simulink model "MOBATSim"  (R2021a)
settings: Solver=FixedStepAuto  StartTime=0.0  StopTime=Sim_t  FixedStep=0.01  MinStep=0.01  RelTol=1e-2
undefined symbols (not defined in the file): meters, Sim_Ts, Vehicle_id, Vehicles
libraries: simulink x31, robotalgslib x11, drivingvehiclecontroller x11, mpcadaslib x1, pid_lib x1
(part 1 of 5)
Description:
  | MOBATSim (Model-based Autonomous Traffic Simulation Framework) is a simulation framework based on MATLAB and Simulink that allows users to develop automated driving algorithms to assess their safety and performance. By running a traffic simulation, the safety of the implemented component or algorithm is measured on both the vehicle level and the traffic level, supported by 2D and 3D visualization options.
settings Model: VariantFading=off  Creator=Mustafa  LastModifiedBy=RanGreidi
settings SolverCC: AlgebraicLoopSolver=TrustRegion  AutoInsertRateTranBlk=on  InsertRTBMode=Always  MinimalZcImpactIntegration=on
settings DataIOCC: ReturnWorkspaceOutputs=off
settings DebuggingCC: AlgebraicLoopMsg=error  UniqueDataStoreMsg=error  SFMachineParentedDataDiag=warning  ArithmeticOperatorsInVariantConditions=warning
settings SFSimCC: SimUseLocalCustomCode=off  CustomCodeUndefinedFunction=UseInterfaceOnly
settings RTWCC: RTWUseLocalCustomCode=off
settings CodeAppCC: StateflowObjectComments=on

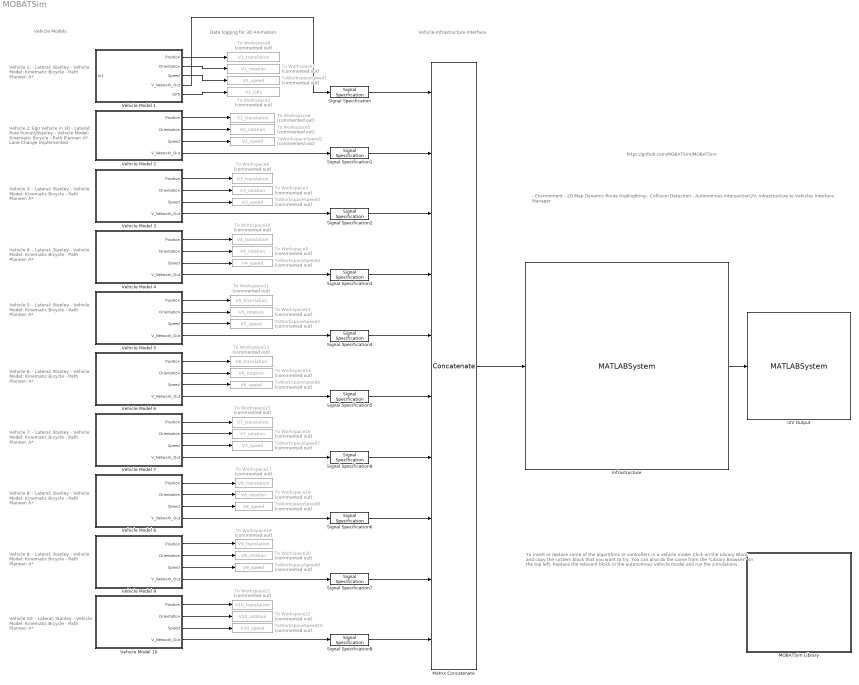
== system MOBATSim ==
  note: Vehicle 1:
      | - Lateral: Stanley
      | - Vehicle Model: Kinematic Bicycle
      | - Path Planner: A*
  note: https://github.com/MOBATSim/MOBATSim
  note: To insert or replace some of the algorithms
      | or controllers in a vehicle mode:
      | Click on the Library Block and copy the system block that you want to try. You can also do the same from the "Library Browser" on the top left.
      | Replace the relevant block in the autonomous vehicle model and run the simulations.
  note: Data logging for 3D Animation
  note: Vehicle-Infrastructure Interface
  note: Vehicle 2: Ego Vehicle in 3D
      | - Lateral: Pure Pursuit/Stanley
      | - Vehicle Model: Kinematic Bicycle
      | - Path Planner: A*
      | - Lane Change Implemented
  note: Vehicle 3:
      | - Lateral: Stanley
      | - Vehicle Model: Kinematic Bicycle
      | - Path Planner: A*
  note: Vehicle 4:
      | - Lateral: Stanley
      | - Vehicle Model: Kinematic Bicycle
      | - Path Planner: A*
  note: Vehicle 6:
      | - Lateral: Stanley
      | - Vehicle Model: Kinematic Bicycle
      | - Path Planner: A*
  note: Vehicle 7:
      | - Lateral: Stanley
      | - Vehicle Model: Kinematic Bicycle
      | - Path Planner: A*
  note: Vehicle 8:
      | - Lateral: Stanley
      | - Vehicle Model: Kinematic Bicycle
      | - Path Planner: A*
  note: Vehicle 9:
      | - Lateral: Stanley
      | - Vehicle Model: Kinematic Bicycle
      | - Path Planner: A*
  note: Vehicle 10:
      | - Lateral: Stanley
      | - Vehicle Model: Kinematic Bicycle
      | - Path Planner: A*
  note: Vehicle 5:
      | - Lateral: Stanley
      | - Vehicle Model: Kinematic Bicycle
      | - Path Planner: A*
  note: Vehicle Models
  note: I2V: Infrastructure to Vehicles Interface
  note: - Environment
      | - 2D Map Dynamic Route Highlighting
      | - Collision Detection
      | - Autonomous Intersection Manager
  I2V Output : MATLABSystem  System=I2V  SimulateUsing=Interpreted execution
      mask Type: I2V
      mask Display:
      | image('MOBATSIM-Icon-Set_3- Flags.png');
      | port_label('input',1,'Flags');
  Infrastructure : MATLABSystem  Description=An instance of the Map.m Class is created.  System=Infrastructure  nrVehicles=length(Vehicles)  SimulateUsing=Interpreted execution
      mask Type: Infrastructure
      mask Display:
      | image('MOBATSIM-Icon-Set_5- Intersection.png');
      | port_label('input',1,'V2Idata');
      | port_label('output',1,'StopCommands');
  MOBATSim Library : Subsystem
      mask Display: image('$imagefile'); % Use "Edit Image" on toolstrip to change.
  Matrix Concatenate : Concatenate  NumInputs=10  Mode=Multidimensional array
  Signal Specification{,1..9} (10 alike) : SignalSpecification  Dimensions=[1 2]
  To Workspace1 : ToWorkspace  Commented=on  VariableName=V1_GPS  SaveFormat=Timeseries  SampleTime=-1
  To Workspace10 : ToWorkspace  Commented=on  VariableName=V4_translation  SaveFormat=Timeseries  SampleTime=-1
  To Workspace11 : ToWorkspace  Commented=on  VariableName=V5_translation  SaveFormat=Timeseries  SampleTime=-1
  To Workspace12 : ToWorkspace  Commented=on  VariableName=V5_rotation  SaveFormat=Timeseries  SampleTime=-1
  To Workspace13 : ToWorkspace  Commented=on  VariableName=V6_translation  SaveFormat=Timeseries  SampleTime=-1
  To Workspace14 : ToWorkspace  Commented=on  VariableName=V6_rotation  SaveFormat=Timeseries  SampleTime=-1
  To Workspace15 : ToWorkspace  Commented=on  VariableName=V7_translation  SaveFormat=Timeseries  SampleTime=-1
  To Workspace16 : ToWorkspace  Commented=on  VariableName=V7_rotation  SaveFormat=Timeseries  SampleTime=-1
  To Workspace17 : ToWorkspace  Commented=on  VariableName=V8_translation  SaveFormat=Timeseries  SampleTime=-1
  To Workspace18 : ToWorkspace  Commented=on  VariableName=V8_rotation  SaveFormat=Timeseries  SampleTime=-1
  To Workspace19 : ToWorkspace  Commented=on  VariableName=V9_translation  SaveFormat=Timeseries  SampleTime=-1
  To Workspace20 : ToWorkspace  Commented=on  VariableName=V9_rotation  SaveFormat=Timeseries  SampleTime=-1
  To Workspace21 : ToWorkspace  Commented=on  VariableName=V10_translation  SaveFormat=Timeseries  SampleTime=-1
  To Workspace22 : ToWorkspace  Commented=on  VariableName=V10_rotation  SaveFormat=Timeseries  SampleTime=-1
  To Workspace3 : ToWorkspace  Commented=on  VariableName=V3_rotation  SaveFormat=Timeseries  SampleTime=-1
  To Workspace4 : ToWorkspace  Commented=on  VariableName=V3_translation  SaveFormat=Timeseries  SampleTime=-1
  To Workspace5 : ToWorkspace  Commented=on  VariableName=V2_rotation  SaveFormat=Timeseries  SampleTime=-1
  To Workspace6 : ToWorkspace  Commented=on  VariableName=V2_translation  SaveFormat=Timeseries  SampleTime=-1
  To Workspace7 : ToWorkspace  Commented=on  VariableName=V1_rotation  SaveFormat=Timeseries  SampleTime=-1
  To Workspace8 : ToWorkspace  Commented=on  VariableName=V1_translation  SaveFormat=Timeseries  SampleTime=-1
  To Workspace9 : ToWorkspace  Commented=on  VariableName=V4_rotation  SaveFormat=Timeseries  SampleTime=-1
  ToWorkspaceSpeed1 : ToWorkspace  Commented=on  VariableName=V1_speed  SaveFormat=Timeseries  SampleTime=-1
  ToWorkspaceSpeed10 : ToWorkspace  Commented=on  VariableName=V10_speed  SaveFormat=Timeseries  SampleTime=-1
  ToWorkspaceSpeed2 : ToWorkspace  Commented=on  VariableName=V2_speed  SaveFormat=Timeseries  SampleTime=-1
  "ToWorkspaceSpeed3 " : ToWorkspace  Commented=on  VariableName=V3_speed  SaveFormat=Timeseries  SampleTime=-1
  ToWorkspaceSpeed4 : ToWorkspace  Commented=on  VariableName=V4_speed  SaveFormat=Timeseries  SampleTime=-1
  ToWorkspaceSpeed5 : ToWorkspace  Commented=on  VariableName=V5_speed  SaveFormat=Timeseries  SampleTime=-1
  ToWorkspaceSpeed6 : ToWorkspace  Commented=on  VariableName=V6_speed  SaveFormat=Timeseries  SampleTime=-1
  ToWorkspaceSpeed7 : ToWorkspace  Commented=on  VariableName=V7_speed  SaveFormat=Timeseries  SampleTime=-1
  ToWorkspaceSpeed8 : ToWorkspace  Commented=on  VariableName=V8_speed  SaveFormat=Timeseries  SampleTime=-1
  ToWorkspaceSpeed9 : ToWorkspace  Commented=on  VariableName=V9_speed  SaveFormat=Timeseries  SampleTime=-1
  Vehicle Model 1 : Subsystem  Description=Tag: Autonomous Vehicle Model  SystemSampleTime=0.01  mask{Vehicle_id=1}
      mask TypeOptions Vehicle_id: MATLAB System2/Vehicle_id
      mask DialogControl DescTextVar Prompt: Autonomous Vehicle Model defined as a system, press the arrow on the lower left corner to see the subsystems. The initial parameters below should be taken from the base workspace but you can edit them anyway you like.
      mask Display: image('$imagefile'); % Use "Edit Image" on toolstrip to change.
  Vehicle Model 10 : Subsystem  Description=Tag: Autonomous Vehicle Model  SystemSampleTime=0.01  mask{Vehicle_id=10}
      mask TypeOptions Vehicle_id: MATLAB System2/Vehicle_id
      mask DialogControl DescTextVar Prompt: Autonomous Vehicle Model defined as a system, press the arrow on the lower left corner to see the subsystems. The initial parameters below should be taken from the base workspace but you can edit them anyway you like.
      mask Display: image('$imagefile'); % Use "Edit Image" on toolstrip to change.
  Vehicle Model 2 : Subsystem  Description=Tag: Autonomous Vehicle Model  SystemSampleTime=0.01  mask{Vehicle_id=2}
      mask TypeOptions Vehicle_id: MATLAB System2/Vehicle_id
      mask DialogControl DescTextVar Prompt: Autonomous Vehicle Model defined as a system, press the arrow on the lower left corner to see the subsystems. The initial parameters below should be taken from the base workspace but you can edit them anyway you like.
      mask Display: image('$imagefile'); % Use "Edit Image" on toolstrip to change.
  Vehicle Model 3 : Subsystem  Description=Tag: Autonomous Vehicle Model  SystemSampleTime=0.01  mask{Vehicle_id=3}
      mask TypeOptions Vehicle_id: MATLAB System2/Vehicle_id
      mask DialogControl DescTextVar Prompt: Autonomous Vehicle Model defined as a system, press the arrow on the lower left corner to see the subsystems. The initial parameters below should be taken from the base workspace but you can edit them anyway you like.
      mask Display: image('$imagefile'); % Use "Edit Image" on toolstrip to change.
  Vehicle Model 4 : Subsystem  Description=Tag: Autonomous Vehicle Model  SystemSampleTime=0.01  mask{Vehicle_id=4}
      mask TypeOptions Vehicle_id: MATLAB System2/Vehicle_id
      mask DialogControl DescTextVar Prompt: Autonomous Vehicle Model defined as a system, press the arrow on the lower left corner to see the subsystems. The initial parameters below should be taken from the base workspace but you can edit them anyway you like.
      mask Display: image('$imagefile'); % Use "Edit Image" on toolstrip to change.
  Vehicle Model 5 : Subsystem  Description=Tag: Autonomous Vehicle Model  SystemSampleTime=0.01  mask{Vehicle_id=5}
      mask TypeOptions Vehicle_id: MATLAB System2/Vehicle_id
      mask DialogControl DescTextVar Prompt: Autonomous Vehicle Model defined as a system, press the arrow on the lower left corner to see the subsystems. The initial parameters below should be taken from the base workspace but you can edit them anyway you like.
      mask Display: image('$imagefile'); % Use "Edit Image" on toolstrip to change.
  Vehicle Model 6 : Subsystem  Description=Tag: Autonomous Vehicle Model  SystemSampleTime=0.01  mask{Vehicle_id=6}
      mask TypeOptions Vehicle_id: MATLAB System2/Vehicle_id
      mask DialogControl DescTextVar Prompt: Autonomous Vehicle Model defined as a system, press the arrow on the lower left corner to see the subsystems. The initial parameters below should be taken from the base workspace but you can edit them anyway you like.
      mask Display: image('$imagefile'); % Use "Edit Image" on toolstrip to change.
  Vehicle Model 7 : Subsystem  Description=Tag: Autonomous Vehicle Model  SystemSampleTime=0.01  mask{Vehicle_id=7}
      mask TypeOptions Vehicle_id: MATLAB System2/Vehicle_id
      mask DialogControl DescTextVar Prompt: Autonomous Vehicle Model defined as a system, press the arrow on the lower left corner to see the subsystems. The initial parameters below should be taken from the base workspace but you can edit them anyway you like.
      mask Display: image('$imagefile'); % Use "Edit Image" on toolstrip to change.
  Vehicle Model 8 : Subsystem  Description=Tag: Autonomous Vehicle Model  SystemSampleTime=0.01  mask{Vehicle_id=8}
      mask TypeOptions Vehicle_id: MATLAB System2/Vehicle_id
      mask DialogControl DescTextVar Prompt: Autonomous Vehicle Model defined as a system, press the arrow on the lower left corner to see the subsystems. The initial parameters below should be taken from the base workspace but you can edit them anyway you like.
      mask Display: image('$imagefile'); % Use "Edit Image" on toolstrip to change.
  Vehicle Model 9 : Subsystem  Description=Tag: Autonomous Vehicle Model  SystemSampleTime=0.01  mask{Vehicle_id=9}
      mask TypeOptions Vehicle_id: MATLAB System2/Vehicle_id
      mask DialogControl DescTextVar Prompt: Autonomous Vehicle Model defined as a system, press the arrow on the lower left corner to see the subsystems. The initial parameters below should be taken from the base workspace but you can edit them anyway you like.
      mask Display: image('$imagefile'); % Use "Edit Image" on toolstrip to change.
  wires:
  Vehicle Model 1/1(Position) -> To Workspace8/1
  Vehicle Model 1/2(Orientation) -> To Workspace7/1
  Vehicle Model 1/4(V_Network_Out) -> Signal Specification/1
  Signal Specification/1 -> Matrix Concatenate/1
  Signal Specification1/1 -> Matrix Concatenate/2
  Vehicle Model 2/2(Orientation) -> To Workspace5/1
  Vehicle Model 2/1(Position) -> To Workspace6/1
  Vehicle Model 3/2(Orientation) -> To Workspace3/1
  Vehicle Model 3/1(Position) -> To Workspace4/1
  Signal Specification2/1 -> Matrix Concatenate/3
  Infrastructure/1 -> I2V Output/1
  Vehicle Model 8/4(V_Network_Out) -> Signal Specification6/1
  Vehicle Model 9/4(V_Network_Out) -> Signal Specification7/1
  Vehicle Model 10/4(V_Network_Out) -> Signal Specification8/1
  Signal Specification3/1 -> Matrix Concatenate/4
  Signal Specification4/1 -> Matrix Concatenate/5
  Signal Specification5/1 -> Matrix Concatenate/6
  Signal Specification9/1 -> Matrix Concatenate/7
  Signal Specification6/1 -> Matrix Concatenate/8
  Signal Specification7/1 -> Matrix Concatenate/9
  Signal Specification8/1 -> Matrix Concatenate/10
  Vehicle Model 4/2(Orientation) -> To Workspace9/1
  Vehicle Model 4/1(Position) -> To Workspace10/1
  Vehicle Model 6/2(Orientation) -> To Workspace14/1
  Vehicle Model 6/1(Position) -> To Workspace13/1
  Vehicle Model 7/2(Orientation) -> To Workspace16/1
  Vehicle Model 7/1(Position) -> To Workspace15/1
  Vehicle Model 8/2(Orientation) -> To Workspace18/1
  Vehicle Model 8/1(Position) -> To Workspace17/1
  Vehicle Model 9/2(Orientation) -> To Workspace20/1
  Vehicle Model 9/1(Position) -> To Workspace19/1
  Vehicle Model 10/2(Orientation) -> To Workspace22/1
  Vehicle Model 10/1(Position) -> To Workspace21/1
  Matrix Concatenate/1 -> Infrastructure/1
  Vehicle Model 2/4(V_Network_Out) -> Signal Specification1/1
  Vehicle Model 3/4(V_Network_Out) -> Signal Specification2/1
  Vehicle Model 4/4(V_Network_Out) -> Signal Specification3/1
  Vehicle Model 6/4(V_Network_Out) -> Signal Specification5/1
  Vehicle Model 7/4(V_Network_Out) -> Signal Specification9/1
  Vehicle Model 5/1(Position) -> To Workspace11/1
  Vehicle Model 5/2(Orientation) -> To Workspace12/1
  Vehicle Model 5/4(V_Network_Out) -> Signal Specification4/1
  Vehicle Model 1/3(Speed) -> ToWorkspaceSpeed1/1
  Vehicle Model 2/3(Speed) -> ToWorkspaceSpeed2/1
  Vehicle Model 3/3(Speed) -> "ToWorkspaceSpeed3 "/1
  Vehicle Model 4/3(Speed) -> ToWorkspaceSpeed4/1
  Vehicle Model 5/3(Speed) -> ToWorkspaceSpeed5/1
  Vehicle Model 6/3(Speed) -> ToWorkspaceSpeed6/1
  Vehicle Model 7/3(Speed) -> ToWorkspaceSpeed7/1
  Vehicle Model 8/3(Speed) -> ToWorkspaceSpeed8/1
  Vehicle Model 9/3(Speed) -> ToWorkspaceSpeed9/1
  Vehicle Model 10/3(Speed) -> ToWorkspaceSpeed10/1
  Vehicle Model 1/5(GPS) -> To Workspace1/1

== system MOBATSim/MOBATSim Library ==
  note: Different pathplanner algorithms with the same input/outputs. Some details and computational performances may differ.
  note: The ACC Classical Block from the MathWorks Example:
      | https://www.mathworks.com/help/driving/examples/adaptive-cruise-control-with-sensor-fusion.html
  note: Path Planners - MATLAB System Blocks
  note: Platoon Controllers - Subsystem Blocks
  note: Platoon controller-PID with a safe distance controller for safely following the
      | leading vehicle. Most vehicles have this block because it is simple and fast
      | in terms of execution time. Can be tuned.
  note: Standard MPC - Adaptive Cruise Control Block. Safest option but computationally
      | expensive. Tradeoff between safety and computational performance depends on
      | the prediction horizon variable.
  note: Lateral Controllers with MATLAB System Blocks
  ACC Classical : Subsystem  Commented=on  TreatAsAtomicUnit=on  VariantControl=controller_type == 1
      settings: RTWFileNameOpts=Use function name
  Adaptive Cruise Control System : mpcadaslib/Adaptive Cruise Control System  Commented=on  EgoModel=tf(1,[1,0])  InitialEgoVelocity=0  DefaultSpacing=Vehicles(Vehicle_id).sensors.safeDistance  MaxVelocity=Vehicles(Vehicle_id).dynamics.maxSpeed  MinAcceleration=-3  amin_ext=off  MaxAcceleration=2  amax_ext=off  Ts=0.1  PredictionHorizon=100  ControllerBehavior=0.620  suboptimal=off  maxiter=10  datatypeopt=double  optmode=off  trackmode=off
  Path Planner - AStar : MATLABSystem  Commented=on  System=VehiclePathPlanner_Astar  Vehicle_id=Vehicle_id  SimulateUsing=Interpreted execution
      mask Type: VehiclePathPlanner_Astar
      mask Display:
      | image('MOBATSIM-Icon-Set_8- Navigation.png');
      | port_label('input',1,'CommunicationIDs');
      | port_label('output',1,'waypointReached');
  Path Planner - Shortest : MATLABSystem  Commented=on  System=VehiclePathPlanner_shortestPathFinder  Vehicle_id=Vehicle_id  SimulateUsing=Interpreted execution
      mask Type: VehiclePathPlanner_shortestPathFinder
      mask Display:
      | image('MOBATSIM-Icon-Set_8- Navigation.png');
      | port_label('input',1,'CommunicationIDs');
      | port_label('output',1,'waypointReached');
  Platoon Controller - PID : Subsystem  Commented=on
  Pure Pursuit with Lane Changing : Subsystem  Commented=on
  Stanley Lateral Control : Subsystem  Commented=on

== system MOBATSim/Vehicle Model 1 ==
  note: Perception
  note: Decision-Making
  note: Control
  In1 : Inport
  Behavioural Planner : MATLABSystem  System=VehicleDrivingMode  Vehicle_id=Vehicle_id  SimulateUsing=Interpreted execution
      mask Type: VehicleDrivingMode
      mask Display:
      | image('MOBATSIM-Icon-Set_7- Behavioural Planner.png');
      | port_label('input',1,'vehicleDetected');
      | port_label('output',1,'SpeedReference');
      | port_label('output',2,'DistanceReference');
      | port_label('output',3,'LeadSpeed');
      | port_label('output',4,'DrivingMode');
      | port_label('output',5,'Dist2Stop');
      | port_label('output',6,'laneChange');
  From Workspace : FromWorkspace  VariableName=Vehicles(1,1).dynamics.GPS  SampleTime=0.02
  Longitudinal and Lateral Controllers : Subsystem
  Safety Filter : Subsystem
  Transform to MOBATSim Coordinates : Subsystem
  Vehicle Model - Kinematic 3DOF Single Track : Subsystem  mask{Vehicle_id=Vehicle_id}
      mask prompts: Vehicle_id "Vehicle ID"
      mask Display: image('MOBATSIM-Icon-Set_13- VehicleModel.png'); % Use "Edit Image" on toolstrip to change.
  Vehicle Path Planner : MATLABSystem  System=VehiclePathPlanner_Astar  Vehicle_id=Vehicle_id  SimulateUsing=Interpreted execution
      mask Type: VehiclePathPlanner_Astar
      mask Display:
      | image('MOBATSIM-Icon-Set_8- Navigation.png');
      | port_label('input',1,'CommunicationIDs');
      | port_label('output',1,'waypointReached');
  Vehicle Sensors : MATLABSystem  System=VehicleSensors  Vehicle_id=Vehicle_id  Tsample=Sim_Ts  OffsetTime=0  SimulateUsing=Interpreted execution
      mask Type: VehicleSensors
      mask Display:
      | image('MOBATSIM-Icon-Set_4- Sensor.png');
      | port_label('output',1,'V2VcommIDs');
      | port_label('output',2,'vehicleDetected');
  Vehicle V2I Output : MATLABSystem  System=VehicleV2I_Out  Vehicle_id=Vehicle_id  SimulateUsing=Interpreted execution
      mask Type: VehicleV2I_Out
      mask Display:
      | image('MOBATSIM-Icon-Set_6- V2l.png');
      | port_label('input',1,'waypointReached');
      | port_label('output',1,'V2Idata');
  Position : Outport  VectorParamsAs1DForOutWhenUnconnected=off
  Orientation : Outport  Port=2  VectorParamsAs1DForOutWhenUnconnected=off
  Speed : Outport  Port=3  VectorParamsAs1DForOutWhenUnconnected=off
  V_Network_Out : Outport  Port=4  VectorParamsAs1DForOutWhenUnconnected=off
  GPS : Outport  Port=5  VectorParamsAs1DForOutWhenUnconnected=off
  wires:
  Vehicle Path Planner/1 -> Vehicle V2I Output/1
  Vehicle Sensors/1 -> Vehicle Path Planner/1
  Vehicle V2I Output/1 -> V_Network_Out/1
  Vehicle Sensors/2 -> Behavioural Planner/1
  Behavioural Planner/1 -> Longitudinal and Lateral Controllers/1(Speed Reference)
  Behavioural Planner/2 -> Longitudinal and Lateral Controllers/2(Inter Vehicular Distance)
  Behavioural Planner/3 -> Longitudinal and Lateral Controllers/3(Lead Speed)
  Behavioural Planner/4 -> Longitudinal and Lateral Controllers/4(drivingMode)
  Behavioural Planner/5 -> Longitudinal and Lateral Controllers/5(Dist2Stop)
  Transform to MOBATSim Coordinates/1(Position) -> Position/1
  Transform to MOBATSim Coordinates/2(Orientation) -> Orientation/1
  Vehicle Model - Kinematic 3DOF Single Track/2(xdot) -> Longitudinal and Lateral Controllers/7(Actual Speed), Speed/1
  Vehicle Model - Kinematic 3DOF Single Track/1(Pose) -> Longitudinal and Lateral Controllers/8(Actual Pose), Transform to MOBATSim Coordinates/1(Pose)
  Longitudinal and Lateral Controllers/1(ref Acc) -> Safety Filter/1(Reference Acceleration)
  Longitudinal and Lateral Controllers/2(ref Steering) -> Safety Filter/2(Reference Steering Angle)
  Safety Filter/1(Steering Angle Cmd) -> Vehicle Model - Kinematic 3DOF Single Track/1(WhlAngF)
  Safety Filter/2(Speed_input) -> Vehicle Model - Kinematic 3DOF Single Track/2(xdotin)
  Behavioural Planner/6 -> Longitudinal and Lateral Controllers/6(laneChange)
  From Workspace/1 -> ?

== system MOBATSim/Vehicle Model 10 ==
  note: Perception
  note: Decision-Making
  note: Control
  Behavioural Planner : MATLABSystem  System=VehicleDrivingMode  Vehicle_id=Vehicle_id  SimulateUsing=Interpreted execution
      mask Type: VehicleDrivingMode
      mask Display:
      | image('MOBATSIM-Icon-Set_7- Behavioural Planner.png');
      | port_label('input',1,'vehicleDetected');
      | port_label('output',1,'SpeedReference');
      | port_label('output',2,'DistanceReference');
      | port_label('output',3,'LeadSpeed');
      | port_label('output',4,'DrivingMode');
      | port_label('output',5,'Dist2Stop');
      | port_label('output',6,'laneChange');
  Longitudinal and Lateral Controllers : Subsystem
  Safety Filter : Subsystem
  Transform to MOBATSim Coordinates : Subsystem
  Vehicle Model - Kinematic 3DOF Single Track : Subsystem  mask{Vehicle_id=Vehicle_id}
      mask prompts: Vehicle_id "Vehicle ID"
      mask Display: image('MOBATSIM-Icon-Set_13- VehicleModel.png'); % Use "Edit Image" on toolstrip to change.
  Vehicle Path Planner : MATLABSystem  System=VehiclePathPlanner_Astar  Vehicle_id=Vehicle_id  SimulateUsing=Interpreted execution
      mask Type: VehiclePathPlanner_Astar
      mask Display:
      | image('MOBATSIM-Icon-Set_8- Navigation.png');
      | port_label('input',1,'CommunicationIDs');
      | port_label('output',1,'waypointReached');
  Vehicle Sensors : MATLABSystem  System=VehicleSensors  Vehicle_id=Vehicle_id  Tsample=Sim_Ts  OffsetTime=0  SimulateUsing=Interpreted execution
      mask Type: VehicleSensors
      mask Display:
      | image('MOBATSIM-Icon-Set_4- Sensor.png');
      | port_label('output',1,'V2VcommIDs');
      | port_label('output',2,'vehicleDetected');
  Vehicle V2I Output : MATLABSystem  System=VehicleV2I_Out  Vehicle_id=Vehicle_id  SimulateUsing=Interpreted execution
      mask Type: VehicleV2I_Out
      mask Display:
      | image('MOBATSIM-Icon-Set_6- V2l.png');
      | port_label('input',1,'waypointReached');
      | port_label('output',1,'V2Idata');
  Position : Outport  VectorParamsAs1DForOutWhenUnconnected=off
  Orientation : Outport  Port=2  VectorParamsAs1DForOutWhenUnconnected=off
  Speed : Outport  Port=3  VectorParamsAs1DForOutWhenUnconnected=off
  V_Network_Out : Outport  Port=4  VectorParamsAs1DForOutWhenUnconnected=off
  wires:
  Vehicle Path Planner/1 -> Vehicle V2I Output/1
  Vehicle Sensors/1 -> Vehicle Path Planner/1
  Vehicle V2I Output/1 -> V_Network_Out/1
  Vehicle Sensors/2 -> Behavioural Planner/1
  Behavioural Planner/1 -> Longitudinal and Lateral Controllers/1(Speed Reference)
  Behavioural Planner/2 -> Longitudinal and Lateral Controllers/2(Inter Vehicular Distance)
  Behavioural Planner/3 -> Longitudinal and Lateral Controllers/3(Lead Speed)
  Behavioural Planner/4 -> Longitudinal and Lateral Controllers/4(drivingMode)
  Behavioural Planner/5 -> Longitudinal and Lateral Controllers/5(Dist2Stop)
  Transform to MOBATSim Coordinates/1(Position) -> Position/1
  Transform to MOBATSim Coordinates/2(Orientation) -> Orientation/1
  Vehicle Model - Kinematic 3DOF Single Track/2(xdot) -> Longitudinal and Lateral Controllers/7(Actual Speed), Speed/1
  Vehicle Model - Kinematic 3DOF Single Track/1(Pose) -> Longitudinal and Lateral Controllers/8(Actual Pose), Transform to MOBATSim Coordinates/1(Pose)
  Longitudinal and Lateral Controllers/1(ref Acc) -> Safety Filter/1(Reference Acceleration)
  Longitudinal and Lateral Controllers/2(ref Steering) -> Safety Filter/2(Reference Steering Angle)
  Safety Filter/1(Steering Angle Cmd) -> Vehicle Model - Kinematic 3DOF Single Track/1(WhlAngF)
  Safety Filter/2(Speed_input) -> Vehicle Model - Kinematic 3DOF Single Track/2(xdotin)
  Behavioural Planner/6 -> Longitudinal and Lateral Controllers/6(laneChange)

== system MOBATSim/Vehicle Model 2 ==
  note: Decision-Making
  note: Control
  note: Perception
  Behavioural Planner - Ego Vehicle : MATLABSystem  System=VehicleDrivingMode_Ego  Vehicle_id=Vehicle_id  SimulateUsing=Interpreted execution
      mask Type: VehicleDrivingMode_Ego
      mask Display:
      | image('MOBATSIM-Icon-Set_7- Behavioural Planner.png');
      | port_label('input',1,'vehicleDetected');
      | port_label('output',1,'SpeedReference');
      | port_label('output',2,'DistanceReference');
      | port_label('output',3,'LeadSpeed');
      | port_label('output',4,'DrivingMode');
      | port_label('output',5,'Dist2Stop');
      | port_label('output',6,'laneChange');
  Longitudinal and Lateral Controllers : Subsystem
  Safety Filter : Subsystem
  Transform to MOBATSim Coordinates : Subsystem
  Vehicle Model - Kinematic 3DOF Single Track : Subsystem  mask{Vehicle_id=Vehicle_id}
      mask prompts: Vehicle_id "Vehicle ID"
      mask Display: image('MOBATSIM-Icon-Set_13- VehicleModel.png'); % Use "Edit Image" on toolstrip to change.
  Vehicle Path Planner : MATLABSystem  System=VehiclePathPlanner_Astar  Vehicle_id=Vehicle_id  SimulateUsing=Interpreted execution
      mask Type: VehiclePathPlanner_Astar
      mask Display:
      | image('MOBATSIM-Icon-Set_8- Navigation.png');
      | port_label('input',1,'CommunicationIDs');
      | port_label('output',1,'waypointReached');
  Vehicle Sensors : MATLABSystem  System=VehicleSensors  Vehicle_id=Vehicle_id  Tsample=Sim_Ts  OffsetTime=0  SimulateUsing=Interpreted execution
      mask Type: VehicleSensors
      mask Display:
      | image('MOBATSIM-Icon-Set_4- Sensor.png');
      | port_label('output',1,'V2VcommIDs');
      | port_label('output',2,'vehicleDetected');
  Vehicle V2I Output : MATLABSystem  System=VehicleV2I_Out  Vehicle_id=Vehicle_id  SimulateUsing=Interpreted execution
      mask Type: VehicleV2I_Out
      mask Display:
      | image('MOBATSIM-Icon-Set_6- V2l.png');
      | port_label('input',1,'waypointReached');
      | port_label('output',1,'V2Idata');
  Position : Outport  VectorParamsAs1DForOutWhenUnconnected=off
  Orientation : Outport  Port=2  VectorParamsAs1DForOutWhenUnconnected=off
  Speed : Outport  Port=3  VectorParamsAs1DForOutWhenUnconnected=off
  V_Network_Out : Outport  Port=4  VectorParamsAs1DForOutWhenUnconnected=off
  wires:
  Vehicle Path Planner/1 -> Vehicle V2I Output/1
  Vehicle V2I Output/1 -> V_Network_Out/1
  Transform to MOBATSim Coordinates/1(Position) -> Position/1
  Transform to MOBATSim Coordinates/2(Orientation) -> Orientation/1
  Behavioural Planner - Ego Vehicle/1 -> Longitudinal and Lateral Controllers/1(Speed Reference)
  Behavioural Planner - Ego Vehicle/2 -> Longitudinal and Lateral Controllers/2(Inter Vehicular Distance)
  Behavioural Planner - Ego Vehicle/3 -> Longitudinal and Lateral Controllers/3(Lead Speed)
  Behavioural Planner - Ego Vehicle/4 -> Longitudinal and Lateral Controllers/4(Driving Mode)
  Behavioural Planner - Ego Vehicle/5 -> Longitudinal and Lateral Controllers/5(Dist2Stop)
  Behavioural Planner - Ego Vehicle/6 -> Longitudinal and Lateral Controllers/6(laneChange)
  Vehicle Model - Kinematic 3DOF Single Track/2(Speed) -> Speed/1, Longitudinal and Lateral Controllers/8(Actual Speed)
  Vehicle Model - Kinematic 3DOF Single Track/1(Pose) -> Transform to MOBATSim Coordinates/1(Pose), Longitudinal and Lateral Controllers/7(Actual Pose)
  Longitudinal and Lateral Controllers/1(Longitudinal Acceleration Cmd) -> Safety Filter/1(Reference Acceleration)
  Longitudinal and Lateral Controllers/2(Reference Steering Angle) -> Safety Filter/2(Reference Steering Angle)
  Safety Filter/2(Steering Angle Cmd) -> Vehicle Model - Kinematic 3DOF Single Track/2(Steering Angle)
  Safety Filter/1(Speed_input) -> Vehicle Model - Kinematic 3DOF Single Track/1(Longitudinal Speed)
  Vehicle Sensors/2 -> Behavioural Planner - Ego Vehicle/1
  Vehicle Sensors/1 -> Vehicle Path Planner/1

== system MOBATSim/Vehicle Model 3 ==
  note: Perception
  note: Decision-Making
  note: Control
  Behavioural Planner : MATLABSystem  System=VehicleDrivingMode  Vehicle_id=Vehicle_id  SimulateUsing=Interpreted execution
      mask Type: VehicleDrivingMode
      mask Display:
      | image('MOBATSIM-Icon-Set_7- Behavioural Planner.png');
      | port_label('input',1,'vehicleDetected');
      | port_label('output',1,'SpeedReference');
      | port_label('output',2,'DistanceReference');
      | port_label('output',3,'LeadSpeed');
      | port_label('output',4,'DrivingMode');
      | port_label('output',5,'Dist2Stop');
      | port_label('output',6,'laneChange');
  Longitudinal and Lateral Controllers : Subsystem
  Safety Filter : Subsystem
  Transform to MOBATSim Coordinates : Subsystem
  Vehicle Model - Kinematic 3DOF Single Track : Subsystem  mask{Vehicle_id=Vehicle_id}
      mask prompts: Vehicle_id "Vehicle ID"
      mask Display: image('MOBATSIM-Icon-Set_13- VehicleModel.png'); % Use "Edit Image" on toolstrip to change.
  Vehicle Path Planner : MATLABSystem  System=VehiclePathPlanner_Astar  Vehicle_id=Vehicle_id  SimulateUsing=Interpreted execution
      mask Type: VehiclePathPlanner_Astar
      mask Display:
      | image('MOBATSIM-Icon-Set_8- Navigation.png');
      | port_label('input',1,'CommunicationIDs');
      | port_label('output',1,'waypointReached');
  Vehicle Sensors : MATLABSystem  System=VehicleSensors  Vehicle_id=Vehicle_id  Tsample=Sim_Ts  OffsetTime=0  SimulateUsing=Interpreted execution
      mask Type: VehicleSensors
      mask Display:
      | image('MOBATSIM-Icon-Set_4- Sensor.png');
      | port_label('output',1,'V2VcommIDs');
      | port_label('output',2,'vehicleDetected');
  Vehicle V2I Output : MATLABSystem  System=VehicleV2I_Out  Vehicle_id=Vehicle_id  SimulateUsing=Interpreted execution
      mask Type: VehicleV2I_Out
      mask Display:
      | image('MOBATSIM-Icon-Set_6- V2l.png');
      | port_label('input',1,'waypointReached');
      | port_label('output',1,'V2Idata');
  Position : Outport  VectorParamsAs1DForOutWhenUnconnected=off
  Orientation : Outport  Port=2  VectorParamsAs1DForOutWhenUnconnected=off
  Speed : Outport  Port=3  VectorParamsAs1DForOutWhenUnconnected=off
  V_Network_Out : Outport  Port=4  VectorParamsAs1DForOutWhenUnconnected=off
  wires:
  Vehicle Path Planner/1 -> Vehicle V2I Output/1
  Vehicle Sensors/1 -> Vehicle Path Planner/1
  Vehicle V2I Output/1 -> V_Network_Out/1
  Vehicle Sensors/2 -> Behavioural Planner/1
  Behavioural Planner/1 -> Longitudinal and Lateral Controllers/1(Speed Reference)
  Behavioural Planner/2 -> Longitudinal and Lateral Controllers/2(Inter Vehicular Distance)
  Behavioural Planner/3 -> Longitudinal and Lateral Controllers/3(Lead Speed)
  Behavioural Planner/4 -> Longitudinal and Lateral Controllers/4(drivingMode)
  Behavioural Planner/5 -> Longitudinal and Lateral Controllers/5(Dist2Stop)
  Transform to MOBATSim Coordinates/1(Position) -> Position/1
  Transform to MOBATSim Coordinates/2(Orientation) -> Orientation/1
  Vehicle Model - Kinematic 3DOF Single Track/2(xdot) -> Longitudinal and Lateral Controllers/7(Actual Speed), Speed/1
  Vehicle Model - Kinematic 3DOF Single Track/1(Pose) -> Longitudinal and Lateral Controllers/8(Actual Pose), Transform to MOBATSim Coordinates/1(Pose)
  Longitudinal and Lateral Controllers/1(ref Acc) -> Safety Filter/1(Reference Acceleration)
  Longitudinal and Lateral Controllers/2(ref Steering) -> Safety Filter/2(Reference Steering Angle)
  Safety Filter/1(Steering Angle Cmd) -> Vehicle Model - Kinematic 3DOF Single Track/1(WhlAngF)
  Safety Filter/2(Speed_input) -> Vehicle Model - Kinematic 3DOF Single Track/2(xdotin)
  Behavioural Planner/6 -> Longitudinal and Lateral Controllers/6(laneChange)

== system MOBATSim/Vehicle Model 4 ==
  note: Perception
  note: Decision-Making
  note: Control
  Behavioural Planner : MATLABSystem  System=VehicleDrivingMode  Vehicle_id=Vehicle_id  SimulateUsing=Interpreted execution
      mask Type: VehicleDrivingMode
      mask Display:
      | image('MOBATSIM-Icon-Set_7- Behavioural Planner.png');
      | port_label('input',1,'vehicleDetected');
      | port_label('output',1,'SpeedReference');
      | port_label('output',2,'DistanceReference');
      | port_label('output',3,'LeadSpeed');
      | port_label('output',4,'DrivingMode');
      | port_label('output',5,'Dist2Stop');
      | port_label('output',6,'laneChange');
  Longitudinal and Lateral Controllers : Subsystem
  Safety Filter : Subsystem
  Transform to MOBATSim Coordinates : Subsystem
  Vehicle Model - Kinematic 3DOF Single Track : Subsystem  mask{Vehicle_id=Vehicle_id}
      mask prompts: Vehicle_id "Vehicle ID"
      mask Display: image('MOBATSIM-Icon-Set_13- VehicleModel.png'); % Use "Edit Image" on toolstrip to change.
  Vehicle Path Planner : MATLABSystem  System=VehiclePathPlanner_Astar  Vehicle_id=Vehicle_id  SimulateUsing=Interpreted execution
      mask Type: VehiclePathPlanner_Astar
      mask Display:
      | image('MOBATSIM-Icon-Set_8- Navigation.png');
      | port_label('input',1,'CommunicationIDs');
      | port_label('output',1,'waypointReached');
  Vehicle Sensors : MATLABSystem  System=VehicleSensors  Vehicle_id=Vehicle_id  Tsample=Sim_Ts  OffsetTime=0  SimulateUsing=Interpreted execution
      mask Type: VehicleSensors
      mask Display:
      | image('MOBATSIM-Icon-Set_4- Sensor.png');
      | port_label('output',1,'V2VcommIDs');
      | port_label('output',2,'vehicleDetected');
  Vehicle V2I Output : MATLABSystem  System=VehicleV2I_Out  Vehicle_id=Vehicle_id  SimulateUsing=Interpreted execution
      mask Type: VehicleV2I_Out
      mask Display:
      | image('MOBATSIM-Icon-Set_6- V2l.png');
      | port_label('input',1,'waypointReached');
      | port_label('output',1,'V2Idata');
  Position : Outport  VectorParamsAs1DForOutWhenUnconnected=off
  Orientation : Outport  Port=2  VectorParamsAs1DForOutWhenUnconnected=off
  Speed : Outport  Port=3  VectorParamsAs1DForOutWhenUnconnected=off
  V_Network_Out : Outport  Port=4  VectorParamsAs1DForOutWhenUnconnected=off
  wires:
  Vehicle Path Planner/1 -> Vehicle V2I Output/1
  Vehicle Sensors/1 -> Vehicle Path Planner/1
  Vehicle V2I Output/1 -> V_Network_Out/1
  Vehicle Sensors/2 -> Behavioural Planner/1
  Behavioural Planner/1 -> Longitudinal and Lateral Controllers/1(Speed Reference)
  Behavioural Planner/2 -> Longitudinal and Lateral Controllers/2(Inter Vehicular Distance)
  Behavioural Planner/3 -> Longitudinal and Lateral Controllers/3(Lead Speed)
  Behavioural Planner/4 -> Longitudinal and Lateral Controllers/4(drivingMode)
  Behavioural Planner/5 -> Longitudinal and Lateral Controllers/5(Dist2Stop)
  Transform to MOBATSim Coordinates/1(Position) -> Position/1
  Transform to MOBATSim Coordinates/2(Orientation) -> Orientation/1
  Vehicle Model - Kinematic 3DOF Single Track/2(xdot) -> Longitudinal and Lateral Controllers/7(Actual Speed), Speed/1
  Vehicle Model - Kinematic 3DOF Single Track/1(Pose) -> Longitudinal and Lateral Controllers/8(Actual Pose), Transform to MOBATSim Coordinates/1(Pose)
  Longitudinal and Lateral Controllers/1(ref Acc) -> Safety Filter/1(Reference Acceleration)
  Longitudinal and Lateral Controllers/2(ref Steering) -> Safety Filter/2(Reference Steering Angle)
  Safety Filter/1(Steering Angle Cmd) -> Vehicle Model - Kinematic 3DOF Single Track/1(WhlAngF)
  Safety Filter/2(Speed_input) -> Vehicle Model - Kinematic 3DOF Single Track/2(xdotin)
  Behavioural Planner/6 -> Longitudinal and Lateral Controllers/6(laneChange)

== system MOBATSim/Vehicle Model 5 ==
  note: Perception
  note: Decision-Making
  note: Control
  Behavioural Planner : MATLABSystem  System=VehicleDrivingMode  Vehicle_id=Vehicle_id  SimulateUsing=Interpreted execution
      mask Type: VehicleDrivingMode
      mask Display:
      | image('MOBATSIM-Icon-Set_7- Behavioural Planner.png');
      | port_label('input',1,'vehicleDetected');
      | port_label('output',1,'SpeedReference');
      | port_label('output',2,'DistanceReference');
      | port_label('output',3,'LeadSpeed');
      | port_label('output',4,'DrivingMode');
      | port_label('output',5,'Dist2Stop');
      | port_label('output',6,'laneChange');
  Longitudinal and Lateral Controllers : Subsystem
  Safety Filter : Subsystem
  Transform to MOBATSim Coordinates : Subsystem
  Vehicle Model - Kinematic 3DOF Single Track : Subsystem  mask{Vehicle_id=Vehicle_id}
      mask prompts: Vehicle_id "Vehicle ID"
      mask Display: image('MOBATSIM-Icon-Set_13- VehicleModel.png'); % Use "Edit Image" on toolstrip to change.
  Vehicle Path Planner : MATLABSystem  System=VehiclePathPlanner_Astar  Vehicle_id=Vehicle_id  SimulateUsing=Interpreted execution
      mask Type: VehiclePathPlanner_Astar
      mask Display:
      | image('MOBATSIM-Icon-Set_8- Navigation.png');
      | port_label('input',1,'CommunicationIDs');
      | port_label('output',1,'waypointReached');
  Vehicle Sensors : MATLABSystem  System=VehicleSensors  Vehicle_id=Vehicle_id  Tsample=Sim_Ts  OffsetTime=0  SimulateUsing=Interpreted execution
      mask Type: VehicleSensors
      mask Display:
      | image('MOBATSIM-Icon-Set_4- Sensor.png');
      | port_label('output',1,'V2VcommIDs');
      | port_label('output',2,'vehicleDetected');
  Vehicle V2I Output : MATLABSystem  System=VehicleV2I_Out  Vehicle_id=Vehicle_id  SimulateUsing=Interpreted execution
      mask Type: VehicleV2I_Out
      mask Display:
      | image('MOBATSIM-Icon-Set_6- V2l.png');
      | port_label('input',1,'waypointReached');
      | port_label('output',1,'V2Idata');
  Position : Outport  VectorParamsAs1DForOutWhenUnconnected=off
  Orientation : Outport  Port=2  VectorParamsAs1DForOutWhenUnconnected=off
  Speed : Outport  Port=3  VectorParamsAs1DForOutWhenUnconnected=off
  V_Network_Out : Outport  Port=4  VectorParamsAs1DForOutWhenUnconnected=off
  wires:
  Vehicle Path Planner/1 -> Vehicle V2I Output/1
  Vehicle Sensors/1 -> Vehicle Path Planner/1
  Vehicle V2I Output/1 -> V_Network_Out/1
  Vehicle Sensors/2 -> Behavioural Planner/1
  Behavioural Planner/1 -> Longitudinal and Lateral Controllers/1(Speed Reference)
  Behavioural Planner/2 -> Longitudinal and Lateral Controllers/2(Inter Vehicular Distance)
  Behavioural Planner/3 -> Longitudinal and Lateral Controllers/3(Lead Speed)
  Behavioural Planner/4 -> Longitudinal and Lateral Controllers/4(drivingMode)
  Behavioural Planner/5 -> Longitudinal and Lateral Controllers/5(Dist2Stop)
  Transform to MOBATSim Coordinates/1(Position) -> Position/1
  Transform to MOBATSim Coordinates/2(Orientation) -> Orientation/1
  Vehicle Model - Kinematic 3DOF Single Track/2(xdot) -> Longitudinal and Lateral Controllers/7(Actual Speed), Speed/1
  Vehicle Model - Kinematic 3DOF Single Track/1(Pose) -> Longitudinal and Lateral Controllers/8(Actual Pose), Transform to MOBATSim Coordinates/1(Pose)
  Longitudinal and Lateral Controllers/1(ref Acc) -> Safety Filter/1(Reference Acceleration)
  Longitudinal and Lateral Controllers/2(ref Steering) -> Safety Filter/2(Reference Steering Angle)
  Safety Filter/1(Steering Angle Cmd) -> Vehicle Model - Kinematic 3DOF Single Track/1(WhlAngF)
  Safety Filter/2(Speed_input) -> Vehicle Model - Kinematic 3DOF Single Track/2(xdotin)
  Behavioural Planner/6 -> Longitudinal and Lateral Controllers/6(laneChange)

== system MOBATSim/Vehicle Model 6 ==
  note: Perception
  note: Decision-Making
  note: Control
  Behavioural Planner : MATLABSystem  System=VehicleDrivingMode  Vehicle_id=Vehicle_id  SimulateUsing=Interpreted execution
      mask Type: VehicleDrivingMode
      mask Display:
      | image('MOBATSIM-Icon-Set_7- Behavioural Planner.png');
      | port_label('input',1,'vehicleDetected');
      | port_label('output',1,'SpeedReference');
      | port_label('output',2,'DistanceReference');
      | port_label('output',3,'LeadSpeed');
      | port_label('output',4,'DrivingMode');
      | port_label('output',5,'Dist2Stop');
      | port_label('output',6,'laneChange');
  Longitudinal and Lateral Controllers : Subsystem
  Safety Filter : Subsystem
  Transform to MOBATSim Coordinates : Subsystem
  Vehicle Model - Kinematic 3DOF Single Track : Subsystem  mask{Vehicle_id=Vehicle_id}
      mask prompts: Vehicle_id "Vehicle ID"
      mask Display: image('MOBATSIM-Icon-Set_13- VehicleModel.png'); % Use "Edit Image" on toolstrip to change.
  Vehicle Path Planner : MATLABSystem  System=VehiclePathPlanner_Astar  Vehicle_id=Vehicle_id  SimulateUsing=Interpreted execution
      mask Type: VehiclePathPlanner_Astar
      mask Display:
      | image('MOBATSIM-Icon-Set_8- Navigation.png');
      | port_label('input',1,'CommunicationIDs');
      | port_label('output',1,'waypointReached');
  Vehicle Sensors : MATLABSystem  System=VehicleSensors  Vehicle_id=Vehicle_id  Tsample=Sim_Ts  OffsetTime=0  SimulateUsing=Interpreted execution
      mask Type: VehicleSensors
      mask Display:
      | image('MOBATSIM-Icon-Set_4- Sensor.png');
      | port_label('output',1,'V2VcommIDs');
      | port_label('output',2,'vehicleDetected');
  Vehicle V2I Output : MATLABSystem  System=VehicleV2I_Out  Vehicle_id=Vehicle_id  SimulateUsing=Interpreted execution
      mask Type: VehicleV2I_Out
      mask Display:
      | image('MOBATSIM-Icon-Set_6- V2l.png');
      | port_label('input',1,'waypointReached');
      | port_label('output',1,'V2Idata');
  Position : Outport  VectorParamsAs1DForOutWhenUnconnected=off
  Orientation : Outport  Port=2  VectorParamsAs1DForOutWhenUnconnected=off
  Speed : Outport  Port=3  VectorParamsAs1DForOutWhenUnconnected=off
  V_Network_Out : Outport  Port=4  VectorParamsAs1DForOutWhenUnconnected=off
  wires:
  Vehicle Path Planner/1 -> Vehicle V2I Output/1
  Vehicle Sensors/1 -> Vehicle Path Planner/1
  Vehicle V2I Output/1 -> V_Network_Out/1
  Vehicle Sensors/2 -> Behavioural Planner/1
  Behavioural Planner/1 -> Longitudinal and Lateral Controllers/1(Speed Reference)
  Behavioural Planner/2 -> Longitudinal and Lateral Controllers/2(Inter Vehicular Distance)
  Behavioural Planner/3 -> Longitudinal and Lateral Controllers/3(Lead Speed)
  Behavioural Planner/4 -> Longitudinal and Lateral Controllers/4(drivingMode)
  Behavioural Planner/5 -> Longitudinal and Lateral Controllers/5(Dist2Stop)
  Transform to MOBATSim Coordinates/1(Position) -> Position/1
  Transform to MOBATSim Coordinates/2(Orientation) -> Orientation/1
  Vehicle Model - Kinematic 3DOF Single Track/2(xdot) -> Longitudinal and Lateral Controllers/7(Actual Speed), Speed/1
  Vehicle Model - Kinematic 3DOF Single Track/1(Pose) -> Longitudinal and Lateral Controllers/8(Actual Pose), Transform to MOBATSim Coordinates/1(Pose)
  Longitudinal and Lateral Controllers/1(ref Acc) -> Safety Filter/1(Reference Acceleration)
  Longitudinal and Lateral Controllers/2(ref Steering) -> Safety Filter/2(Reference Steering Angle)
  Safety Filter/1(Steering Angle Cmd) -> Vehicle Model - Kinematic 3DOF Single Track/1(WhlAngF)
  Safety Filter/2(Speed_input) -> Vehicle Model - Kinematic 3DOF Single Track/2(xdotin)
  Behavioural Planner/6 -> Longitudinal and Lateral Controllers/6(laneChange)

== system MOBATSim/Vehicle Model 7 ==
  note: Perception
  note: Decision-Making
  note: Control
  Behavioural Planner : MATLABSystem  System=VehicleDrivingMode  Vehicle_id=Vehicle_id  SimulateUsing=Interpreted execution
      mask Type: VehicleDrivingMode
      mask Display:
      | image('MOBATSIM-Icon-Set_7- Behavioural Planner.png');
      | port_label('input',1,'vehicleDetected');
      | port_label('output',1,'SpeedReference');
      | port_label('output',2,'DistanceReference');
      | port_label('output',3,'LeadSpeed');
      | port_label('output',4,'DrivingMode');
      | port_label('output',5,'Dist2Stop');
      | port_label('output',6,'laneChange');
  Longitudinal and Lateral Controllers : Subsystem
  Safety Filter : Subsystem
  Transform to MOBATSim Coordinates : Subsystem
  Vehicle Model - Kinematic 3DOF Single Track : Subsystem  mask{Vehicle_id=Vehicle_id}
      mask prompts: Vehicle_id "Vehicle ID"
      mask Display: image('MOBATSIM-Icon-Set_13- VehicleModel.png'); % Use "Edit Image" on toolstrip to change.
  Vehicle Path Planner : MATLABSystem  System=VehiclePathPlanner_Astar  Vehicle_id=Vehicle_id  SimulateUsing=Interpreted execution
      mask Type: VehiclePathPlanner_Astar
      mask Display:
      | image('MOBATSIM-Icon-Set_8- Navigation.png');
      | port_label('input',1,'CommunicationIDs');
      | port_label('output',1,'waypointReached');
  Vehicle Sensors : MATLABSystem  System=VehicleSensors  Vehicle_id=Vehicle_id  Tsample=Sim_Ts  OffsetTime=0  SimulateUsing=Interpreted execution
      mask Type: VehicleSensors
      mask Display:
      | image('MOBATSIM-Icon-Set_4- Sensor.png');
      | port_label('output',1,'V2VcommIDs');
      | port_label('output',2,'vehicleDetected');
  Vehicle V2I Output : MATLABSystem  System=VehicleV2I_Out  Vehicle_id=Vehicle_id  SimulateUsing=Interpreted execution
      mask Type: VehicleV2I_Out
      mask Display:
      | image('MOBATSIM-Icon-Set_6- V2l.png');
      | port_label('input',1,'waypointReached');
      | port_label('output',1,'V2Idata');
  Position : Outport  VectorParamsAs1DForOutWhenUnconnected=off
  Orientation : Outport  Port=2  VectorParamsAs1DForOutWhenUnconnected=off
  Speed : Outport  Port=3  VectorParamsAs1DForOutWhenUnconnected=off
  V_Network_Out : Outport  Port=4  VectorParamsAs1DForOutWhenUnconnected=off
  wires:
  Vehicle Path Planner/1 -> Vehicle V2I Output/1
  Vehicle Sensors/1 -> Vehicle Path Planner/1
  Vehicle V2I Output/1 -> V_Network_Out/1
  Vehicle Sensors/2 -> Behavioural Planner/1
  Behavioural Planner/1 -> Longitudinal and Lateral Controllers/1(Speed Reference)
  Behavioural Planner/2 -> Longitudinal and Lateral Controllers/2(Inter Vehicular Distance)
  Behavioural Planner/3 -> Longitudinal and Lateral Controllers/3(Lead Speed)
  Behavioural Planner/4 -> Longitudinal and Lateral Controllers/4(drivingMode)
  Behavioural Planner/5 -> Longitudinal and Lateral Controllers/5(Dist2Stop)
  Transform to MOBATSim Coordinates/1(Position) -> Position/1
  Transform to MOBATSim Coordinates/2(Orientation) -> Orientation/1
  Vehicle Model - Kinematic 3DOF Single Track/2(xdot) -> Longitudinal and Lateral Controllers/7(Actual Speed), Speed/1
  Vehicle Model - Kinematic 3DOF Single Track/1(Pose) -> Longitudinal and Lateral Controllers/8(Actual Pose), Transform to MOBATSim Coordinates/1(Pose)
  Longitudinal and Lateral Controllers/1(ref Acc) -> Safety Filter/1(Reference Acceleration)
  Longitudinal and Lateral Controllers/2(ref Steering) -> Safety Filter/2(Reference Steering Angle)
  Safety Filter/1(Steering Angle Cmd) -> Vehicle Model - Kinematic 3DOF Single Track/1(WhlAngF)
  Safety Filter/2(Speed_input) -> Vehicle Model - Kinematic 3DOF Single Track/2(xdotin)
  Behavioural Planner/6 -> Longitudinal and Lateral Controllers/6(laneChange)
